simulink model "odqsim_fbiq"  (R2016b)
settings: Solver=FixedStepDiscrete  StartTime=0.0  StopTime=10.0  FixedStep=Ts  RelTol=1e-3
values from neighbouring files (symbols this model uses):
  K = odqdata.K    [odqlab_interact.m]
  P = odqdata.P    [odqlab_interact.m]
  Q = odqanly(G)    [odq.m]    (also in odqlab_interact.m = odqdata.Q; odqlab_verify.m = odqdata.Q; odqreal.m = orderfields(Q); odqsim.m = varargin{2})
undefined symbols (not defined in the file or in its folder): Ts
libraries: odqblock x5
settings Model: Creator=morita  LastModifiedBy=morita

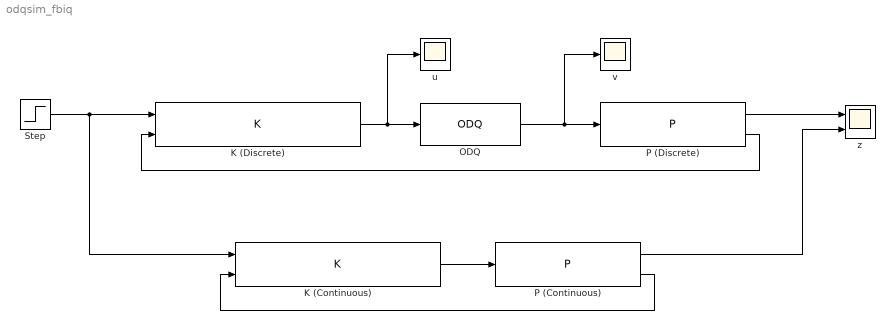
== system odqsim_fbiq ==
  K (Continuous) : odqblock/K  A=K.a  B1=K.b1  B2=K.b2  C=K.c  D1=K.d1  D2=K.d2  Ts=Ts  x0=x0
  K (Discrete) : odqblock/K  A=K.a  B1=K.b1  B2=K.b2  C=K.c  D1=K.d1  D2=K.d2  Ts=Ts  x0=x0
  ODQ : odqblock/ODQ  A=Q.a  B1=Q.b1  B2=Q.b2  C=Q.c  d=d  Ts=Ts
  P (Continuous) : odqblock/P  A=P.a  B=P.b  C1=P.c1  C2=P.c2  Ts=Ts  x0=x0
  P (Discrete) : odqblock/P  A=P.a  B=P.b  C1=P.c1  C2=P.c2  Ts=Ts  x0=x0
  Step : Step  Time=0  SampleTime=0
  u : Scope
  v : Scope
  z : Scope  NumInputPorts=2
  wires:
  K (Continuous)/1 -> P (Continuous)/1
  K (Discrete)/1 -> u/1, ODQ/1
  ODQ/1 -> v/1, P (Discrete)/1
  P (Continuous)/2 -> K (Continuous)/2
  P (Continuous)/1 -> z/2
  P (Discrete)/2 -> K (Discrete)/2
  Step/1 -> K (Continuous)/1, K (Discrete)/1
  P (Discrete)/1 -> z/1
